simulink subsystem "StudentTemplate_ALSILO001_M1"  (R2025a)
settings: Solver=VariableStepAuto  StartTime=0.0  StopTime=10.0  RelTol=1e-3
libraries: cstblocks x4, dspstat3 x1, slpidlib x1, simulink x1
settings Model: Creator=JesseJabezArendse  LastModifiedBy=ilokealusala

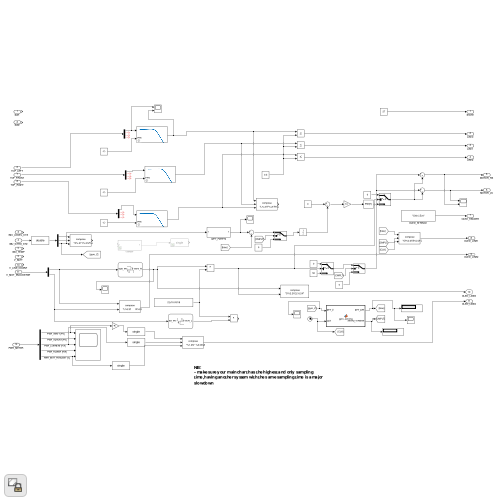
[thumbnail: Simulink's stored preview of the top-level diagram]
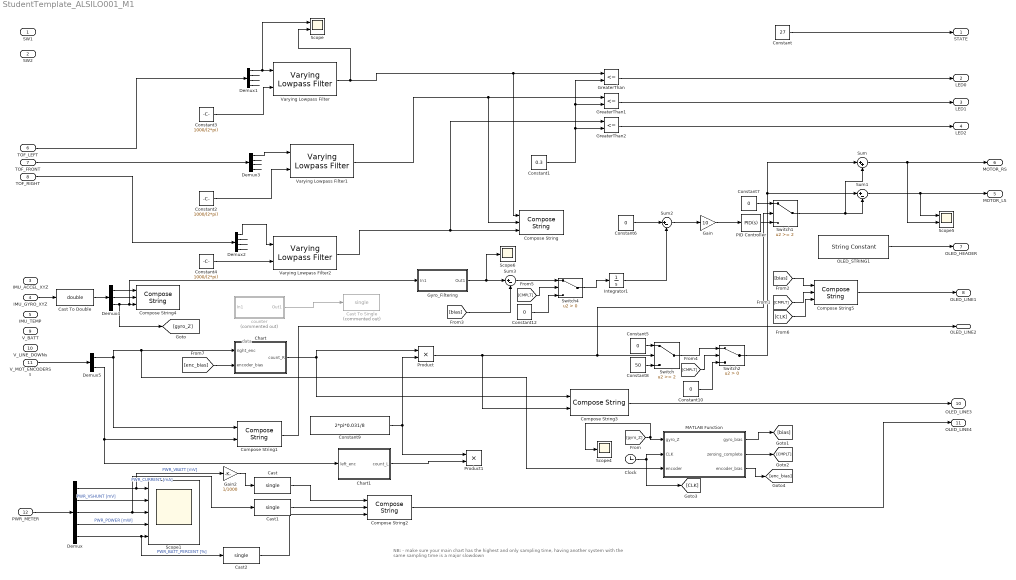
== system StudentTemplate_ALSILO001_M1 ==
  note: data
  note: NB:
      | - make sure your main chart has the highest and only sampling time, having another system with the same sampling time is a major slowdown
  SW1 : Inport
  SW2 : Inport  Port=2
  IMU_ACCEL_XYZ : Inport  Port=3
  IMU_GYRO_XYZ : Inport  Port=4
  IMU_TEMP : Inport  Port=5
  TOF_LEFT : Inport  Port=6
  TOF_FRONT : Inport  Port=7
  TOF_RIGHT : Inport  Port=8
  V_BATT : Inport  Port=9
  V_LINE_DOWNs : Inport  Port=10
  V_MOT_ENCODERSs : Inport  Port=11
  PWR_METER : Inport  Port=12
  Cast : DataTypeConversion  OutDataTypeStr=single  SaturateOnIntegerOverflow=off  RndMeth=Floor
  Cast To Double : DataTypeConversion  OutDataTypeStr=double  SaturateOnIntegerOverflow=off  RndMeth=Floor
  Cast To Single : DataTypeConversion  Commented=on  OutDataTypeStr=single  SaturateOnIntegerOverflow=off  RndMeth=Floor
  Cast1 : DataTypeConversion  OutDataTypeStr=single  SaturateOnIntegerOverflow=off  RndMeth=Floor
  Cast2 : DataTypeConversion  OutDataTypeStr=single  SaturateOnIntegerOverflow=off  RndMeth=Floor
  Chart : Stateflow chart  TreatAsAtomicUnit=on
  Chart1 : Stateflow chart  TreatAsAtomicUnit=on
  Clock : Clock
  Compose String : ComposeString  Format="\"L%.2f F%.2f R%.2f\""
  Compose String1 : ComposeString  Format="\"L%2.2f       R%2.2f f\""
  Compose String2 : ComposeString  Format="\"%1.2fV  %3.0fmA  %2.0f%%\""
  Compose String3 : ComposeString  Format="\"D%2.2f EL%2.0f\""
  Compose String4 : ComposeString  Format="\"X%.2f Y%.2f Z%.2f\""
  Compose String5 : ComposeString  Format="\"Of%2.2f B%2.2f C%2.2f\""
  Constant : Constant  Value=27
  Constant1 : Constant  Value=0.3  SampleTime=-1
  Constant{5..7,10,12} (5 alike) : Constant  Value=0
  Constant2 : Constant  Value=1000/(2*pi)
  Constant3 : Constant  Value=1000/(2*pi)
  Constant4 : Constant  Value=1000/(2*pi)
  Constant8 : Constant  Value=50
  Constant9 : Constant  Value=2*pi*0.031/8
  Demux : Demux  Outputs=5
  Demux1 : Demux
  Demux2 : Demux
  Demux3 : Demux
  Demux4 : Demux  Outputs=3
  Demux5 : Demux  Outputs=2
  Gain : Gain  Gain=10
  Gain2 : Gain  Gain=1/1000
  GreaterThan : RelationalOperator  Operator=<=  OutDataTypeStr=boolean  RndMeth=Simplest  InputSameDT=off
  GreaterThan1 : RelationalOperator  Operator=<=  OutDataTypeStr=boolean  RndMeth=Simplest  InputSameDT=off
  GreaterThan2 : RelationalOperator  Operator=<=  OutDataTypeStr=boolean  RndMeth=Simplest  InputSameDT=off
  Gyro_Filtering : Subsystem
  Integrator1 : Integrator
  MATLAB Function : MATLAB Function  TreatAsAtomicUnit=on
  OLED_STRING1 : StringConstant  String="\"Chini_Evo\""
  PID Controller : slpidlib/PID Controller  Controller=PID  Form=Parallel  TimeDomain=Continuous-time  UseExternalTs=off  SampleTime=-1  IntegratorMethod=Forward Euler  FilterMethod=Forward Euler  ControllerParametersSource=internal  P=1  I=1  UseKiTs=on  D=0  UseExternalDerivativeSource=off  N=100  UseFilter=on  TunerSelectOption=Transfer Function Based (PID Tuner App)  InitialConditionSource=internal  InitialConditionForIntegrator=0  InitialConditionForFilter=0  DifferentiatorICPrevScaledInput=0  ExternalReset=none  TrackingMode=off  Kt=1  LimitOutput=off  SatLimitsSource=internal  UpperSaturationLimit=inf  LowerSaturationLimit=-inf  LinearizeAsGain=on  AntiWindupMode=none  Kb=1  LimitIntegrator=off  UpperIntegratorSaturationLimit=inf  LowerIntegratorSaturationLimit=-inf  POutMin=[]  POutMax=[]  IOutMin=[]  IOutMax=[]  DOutMin=[]  DOutMax=[]  NOutMin=[]  NOutMax=[]  SumOutMin=[]  SumOutMax=[]  SaturationOutMin=[]  SaturationOutMax=[]  PParamMin=[]  PParamMax=[]  IParamMin=[]  IParamMax=[]  DParamMin=[]  DParamMax=[]  NParamMin=[]  NParamMax=[]  KbParamMin=[]  KbParamMax=[]  KtParamMin=[]  KtParamMax=[]  KbOutMin=[]  KbOutMax=[]  KtOutMin=[]  KtOutMax=[]  IntegratorOutMin=[]  IntegratorOutMax=[]  FilterOutMin=[]  FilterOutMax=[]  SumI1OutMin=[]  SumI1OutMax=[]  SumI2OutMin=[]  SumI2OutMax=[]  SumI3OutMin=[]  SumI3OutMax=[]  SumI4OutMin=[]  SumI4OutMax=[]  SumDOutMin=[]  SumDOutMax=[]  DifferentiatorOutMin=[]  DifferentiatorOutMax=[]  FilterDiffOutCoefMin=[]  FilterDiffOutCoefMax=[]  ReciprocalOutMin=[]  ReciprocalOutMax=[]  SumDenOutMin=[]  SumDenOutMax=[]  SumNumOutMin=[]  SumNumOutMax=[]  DivideOutMin=[]  DivideOutMax=[]  UdiffTsProdOutMin=[]  UdiffTsProdOutMax=[]  NTsProdOutMin=[]  NTsProdOutMax=[]  UintegralTsProdOutMin=[]  UintegralTsProdOutMax=[]  UngainTsProdOutMin=[]  UngainTsProdOutMax=[]  ClampingZeroOutDataTypeStr=Inherit: Inherit via back propagation  ClampingZeroOutMin=[]  ClampingZeroOutMax=[]  FilterDenConstantOutDataTypeStr=Inherit: Inherit via back propagation  FilterDenConstantOutMin=[]  FilterDenConstantOutMax=[]  PCopyOutDataTypeStr=Inherit: Inherit via back propagation  PCopyOutMin=[]  PCopyOutMax=[]  NCopyOutDataTypeStr=Inherit: Inherit via back propagation  NCopyOutMin=[]  NCopyOutMax=[]  IntegratorContinuousStateAttributes=''  IntegratorStateMustResolveToSignalObject=off  IntegratorRTWStateStorageClass=Auto  FilterContinuousStateAttributes=''  FilterStateMustResolveToSignalObject=off  FilterRTWStateStorageClass=Auto  ParallelPVariant=InternalParameters  IdealPVariant=Disabled  IVariant=InternalParameters  DVariant=InternalParameters  IntegratorVariant=Continuous  SatVariant=Disabled  AWVariant=Passthrough  PCopyVariant=Disabled  TRVariant=Disabled  FdbkBlocksVariant=Forward  IdealPFdbkVariant=Disabled  SatFdbkVariant=Disabled  DerivativeFilterVariant=ContFilter  NVariant=InternalParameters  NCopyVariant=Disabled  FilterICVariant=InternalICsFilter  IntegratorICVariant=InternalICs  ExternalResetVariant=Disabled  TRSumVariant=Passthrough  SumFdbkVariant=Disabled  SumVariant=Sum_PID  TsampFilterVariant=InternalTs  TsampNgainVariant=Passthrough  TsampIntegralVariant=Disabled_SignalSpec  ExternalSaturationOutDataTypeStr=Inherit: Same as second input  DerivativeSourceVariant=ErrorSignal  PreIntVariant=InternalPreInt
  Product : Product
  Product1 : Product
  Scope : Scope  NumInputPorts=2
      settings: ActiveDisplayYMinimum=0.22759  ActiveDisplayYMaximum=0.52326
  Scope1 : Scope  NumInputPorts=5
      settings: ActiveDisplayYMinimum=-437.5  ActiveDisplayYMaximum=3937.5  DataLoggingVariableName=ScopeData3
  Scope4 : Scope
      settings: ActiveDisplayYMinimum=-1  ActiveDisplayYMaximum=1  DataLoggingVariableName=ScopeData4
  Scope5 : Scope  NumInputPorts=2
      settings: ActiveDisplayYMinimum=-50.220242020461733  ActiveDisplayYMaximum=86.425407854450555  DataLoggingVariableName=ScopeData5
  Scope6 : Scope
      settings: ActiveDisplayYMinimum=-1  ActiveDisplayYMaximum=1  DataLoggingVariableName=ScopeData6
  Sum : Sum  Inputs=|++
  Sum1 : Sum  Inputs=|+-
  Sum2 : Sum  Inputs=|+-
  Sum3 : Sum  Inputs=|+-
  Switch : Switch  Threshold=2  SaturateOnIntegerOverflow=off  InputSameDT=off
  Switch1 : Switch  Threshold=2  SaturateOnIntegerOverflow=off  InputSameDT=off
  Switch2 : Switch  Criteria=u2 > Threshold  SaturateOnIntegerOverflow=off  InputSameDT=off
  Switch4 : Switch  Criteria=u2 > Threshold  SaturateOnIntegerOverflow=off  InputSameDT=off
  Varying Lowpass Filter : cstblocks/Linear Parameter Varying/Varying Lowpass Filter  N=1
  Varying Lowpass Filter1 : cstblocks/Linear Parameter Varying/Varying Lowpass Filter  N=1
  Varying Lowpass Filter2 : cstblocks/Linear Parameter Varying/Varying Lowpass Filter  N=1
  counter : Subsystem  Commented=on
  STATE : Outport
  LED0 : Outport  Port=2
  LED1 : Outport  Port=3
  LED2 : Outport  Port=4
  MOTOR_LS : Outport  Port=5
  MOTOR_RS : Outport  Port=6
  OLED_HEADER : Outport  Port=7
  OLED_LINE1 : Outport  Port=8
  OLED_LINE2 : Outport  Port=9
  OLED_LINE3 : Outport  Port=10
  OLED_LINE4 : Outport  Port=11
  wires:
  TOF_FRONT/1 -> Demux3/1
  Demux2/1 -> Varying Lowpass Filter2/1
  Demux2/3 -> ?
  Demux2/2 -> ?
  Demux2/4 -> ?
  Compose String1/1 -> OLED_LINE2/1
  Varying Lowpass Filter1/1 -> Compose String/2, GreaterThan1/1
  GreaterThan1/1 -> LED1/1
  Constant3/1 -> Varying Lowpass Filter/2
  Demux3/3 -> ?
  TOF_RIGHT/1 -> Demux2/1
  Demux3/4 -> ?
  Demux3/2 -> ?
  Demux1/2 -> ?
  Demux3/1 -> Varying Lowpass Filter1/1
  OLED_STRING1/1 -> OLED_HEADER/1
  Demux1/1 -> Varying Lowpass Filter/1, Scope/1
  Constant1/1 -> GreaterThan2/2, GreaterThan1/2, GreaterThan/2
  Demux1/4 -> ?
  GreaterThan2/1 -> LED2/1
  TOF_LEFT/1 -> Demux1/1
  GreaterThan/1 -> LED0/1
  Demux1/3 -> ?
  PWR_METER/1 -> Demux/1
  Demux/1 -> Scope1/1, Gain2/1  "PWR_VBATT [mV]"
  Demux/2 -> Scope1/2  "PWR_VSHUNT [mV]"
  Demux/3 -> Scope1/3, Cast1/1  "PWR_CURRENT [mA]"
  Demux/4 -> Scope1/4  "PWR_POWER [mW]"
  Demux/5 -> Scope1/5, Cast2/1  "PWR_BATT_PERCENT [%]"
  Compose String2/1 -> OLED_LINE4/1
  Gain2/1 -> Cast/1
  Cast/1 -> Compose String2/1
  Cast1/1 -> Compose String2/2
  Cast2/1 -> Compose String2/3
  Varying Lowpass Filter2/1 -> Compose String/3, GreaterThan2/1
  Varying Lowpass Filter/1 -> Compose String/1, GreaterThan/1, Scope/2
  Constant/1 -> STATE/1
  Constant2/1 -> Varying Lowpass Filter1/2
  Constant4/1 -> Varying Lowpass Filter2/2
  V_MOT_ENCODERSs/1 -> Demux5/1
  Compose String3/1 -> OLED_LINE3/1
  Demux5/2 -> Compose String1/2, Chart1/1(left_enc)
  IMU_GYRO_XYZ/1 -> Cast To Double/1
  Demux4/1 -> Compose String4/1
  Demux4/2 -> Compose String4/2
  Demux4/3 -> Compose String4/3, Gyro_Filtering/1(In1), [gyro_Z]
  Constant6/1 -> Sum2/1
  Sum2/1 -> Gain/1
  PID Controller/1 -> Switch1/3
  Switch1/1 -> Sum/2, Sum1/2
  Constant5/1 -> Switch/1
  Constant8/1 -> Switch/3
  Constant7/1 -> Switch1/1
  Integrator1/1 -> Sum2/2
  Cast To Double/1 -> Demux4/1
  Chart1/1(count_L) -> Product1/2
  Constant9/1 -> Product/2, Product1/1
  Product/1 -> Switch/2, Switch1/2, Compose String3/2
  Clock/1 -> MATLAB Function/2(CLK), [CLK]
  [gyro_Z] -> MATLAB Function/1(gyro_Z), Scope4/1
  MATLAB Function/1(gyro_bias) -> [bias]
  MATLAB Function/2(zeroing_complete) -> [CMPLT]
  Compose String5/1 -> OLED_LINE1/1
  [CMPLT] -> Compose String5/2
  [bias] -> Compose String5/1
  [bias] -> Sum3/2
  Sum3/1 -> Switch4/1
  Switch4/1 -> Integrator1/1
  [CMPLT] -> Switch4/2
  Constant12/1 -> Switch4/3
  Switch2/1 -> Sum1/1, Sum/1
  Switch/1 -> Switch2/1
  [CMPLT] -> Switch2/2
  Constant10/1 -> Switch2/3
  Gain/1 -> PID Controller/1
  [CLK] -> Compose String5/3
  Sum/1 -> MOTOR_RS/1, Scope5/2
  Chart/1(count_R) -> Compose String3/1, Product/1
  Demux5/1 -> Compose String1/1, Chart/1(right_enc), MATLAB Function/3(encoder)
  counter/1(Out1) -> Cast To Single/1
  Sum1/1 -> MOTOR_LS/1, Scope5/1
  Gyro_Filtering/1(Out1) -> Sum3/1, Scope6/1
  MATLAB Function/3(encoder_bias) -> [enc_bias]
  [enc_bias] -> Chart/2(encoder_bias)

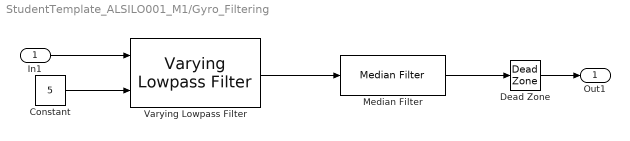
== system StudentTemplate_ALSILO001_M1/Gyro_Filtering ==
  In1 : Inport
  Constant : Constant  Value=5
  Dead Zone : DeadZone  LowerValue=-0.01  UpperValue=0.01
  Median Filter : dspstat3/Median Filter  WindowLength=5  SimulateUsing=Interpreted execution
      settings: LibrarySourceBlock=|
      | dspfdesign/Median
      | Filter
  Varying Lowpass Filter : cstblocks/Linear Parameter Varying/Varying Lowpass Filter  N=1
  Out1 : Outport
  wires:
  Dead Zone/1 -> Out1/1
  In1/1 -> Varying Lowpass Filter/1
  Median Filter/1 -> Dead Zone/1
  Varying Lowpass Filter/1 -> Median Filter/1
  Constant/1 -> Varying Lowpass Filter/2

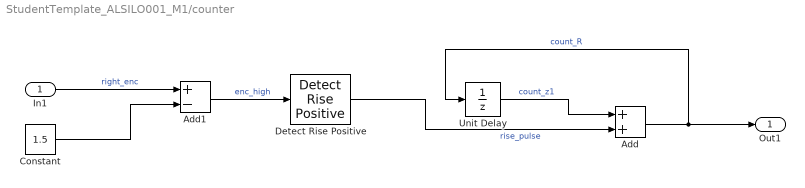
== system StudentTemplate_ALSILO001_M1/counter ==
  In1 : Inport
  Add : Sum
  Add1 : Sum  Inputs=+-
  Constant : Constant  Value=1.5
  Detect Rise Positive : simulink/Logic and Bit Operations/Detect Rise Positive  vinit=0  OutDataTypeStr=uint8
  Unit Delay : UnitDelay  SampleTime=-1  HasFrameUpgradeWarning=on
  Out1 : Outport
  wires:
  Add/1 -> Out1/1, Unit Delay/1  "count_R"
  Unit Delay/1 -> Add/1  "count_z1"
  Detect Rise Positive/1 -> Add/2  "rise_pulse"
  Add1/1 -> Detect Rise Positive/1  "enc_high"
  Constant/1 -> Add1/2
  In1/1 -> Add1/1  "right_enc"

== stateflow chart StudentTemplate_ALSILO001_M1/Chart1 ==
  state PulseDetected
    entry:
    count_L=count_L+1
  state NoPulse
  (default) -> NoPulse : {count_L=0;}
  NoPulse -> PulseDetected : [left_enc>1.5]
  PulseDetected -> NoPulse : [left_enc<1.5]
  data: left_enc input; count_L output

== matlab function StudentTemplate_ALSILO001_M1/MATLAB Function ==
  settings: updateMethod=DISCRETE
  data: gyro_Z input; CLK input; gyro_bias output; zeroing_complete output; encoder input; encoder_bias output
function [gyro_bias, zeroing_complete, encoder_bias]     = gyro_zeroing(gyro_Z, CLK, encoder)
persistent sample_count;
persistent p_gyro_bias;        % Add this - gyro_bias needs to be persistent
persistent enc_bias;

if isempty(sample_count)
    sample_count=0;
    p_gyro_bias=0;
    enc_bias=0;
end
if CLK<0.5
    zeroing_complete=0;
    p_gyro_bias=0;
    gyro_bias=0;
    encoder_bias=0;
    enc_bias=0;
    return
end
if sample_count<1000
    sample_count=sample_count+1;
    p_gyro_bias=(p_gyro_bias+gyro_Z);
    zeroing_complete=0;
    gyro_bias=0;
    encoder_bias=0;
    enc_bias = enc_bias+encoder;
else
    zeroing_complete=1;
    gyro_bias=p_gyro_bias/sample_count;
    encoder_bias = enc_bias/sample_count;
end

== stateflow chart StudentTemplate_ALSILO001_M1/Chart ==
  state NoPulse
  state PulseDetected
    entry:
    count_R = count_R + 1;
    if (right_enc > enc_max)
    enc_max = right_enc;
    end
  (default) -> NoPulse : {
      | count_R=0;
      | enc_max=0;
      | }
  NoPulse -> PulseDetected : [right_enc>(enc_max+encoder_bias)/2]
  PulseDetected -> NoPulse : [right_enc<(enc_max+encoder_bias)/2]
  data: right_enc input; count_R output; encoder_bias input; enc_max local
